simulink model "all_Challenges_all_controllers_slrd"  (R2024a)
settings: Solver=FixedStepAuto  StartTime=0.0  StopTime=inf  RelTol=1e-3  EnableMultiTasking=on
model workspace (MATLAB code in the model file):
  | num_pol_pairs = 7;
  | res_period = 5000;
  | res_pwm   = 2^8;
  | 
  | whl.rad = 0.045;
  | axle.length=0.18;
undefined symbols (not defined in the file): DiscIntNeverNeededParam
libraries: MecRoKa_SFunction_Library x20, slpidlib x5, simulink x4
(part 2 of 2)

== system all_Challenges_all_controllers_slrd/state control/do_BLDC_control.my_control_BLDC2/Task3/Subsystem ==
  Input : Inport
  Inport : Inport  Port=2
  Sum : Sum  Inputs=-+
  Output : Outport
  wires:
  Sum/1 -> Output/1
  Inport/1 -> Sum/1
  Input/1 -> Sum/2

== stateflow chart all_Challenges_all_controllers_slrd/state control ==
  state system_off
    en, du: phi_dot_left   = double(0.0);
    en, du: phi_dot_right = double(0.0);
    en, du: BLDC_on_flag = false;
  state do_BLDC_control
    en, du: BLDC_on_flag = true;
    en, du : [phi_dot_left, phi_dot_right,position_x,yaw_pos,Yaw_rate]=my_control_BLDC2(pitch_est, pitch_rate_est, vel_trgt, yaw_rate_trgt,position_trg,yaw_rate,control_switch,gain_switch);
    state [phi_dot_left1,phi_dot_right1,position_x,yaw_pos,Yaw_rate] = my_control_BLDC2(pitch_est1,pitch_rate_est_in1,vel_trgt_in1,yaw_rate_trgt_in,position_trg,yaw_rate,control_switch,gain_switch) [function]
  (default) -> system_off
  system_off -> do_BLDC_control : [op_mode ~= 0 ]
  do_BLDC_control -> system_off : [op_mode == 0 ]
  data: pitch_est1 function_input double size=1; pitch_rate_est_in1 function_input double size=1; vel_trgt_in1 function_input double size=1; yaw_rate_trgt_in function_input double size=1; phi_dot_left1 function_output double size=1; phi_dot_right1 function_output double size=1; position_trg function_input double size=1; position_x function_output; yaw_rate function_input double size=1; yaw_pos function_output; control_switch function_input double size=1; Yaw_rate function_output; gain_switch function_input double size=1; BLDC_on_flag output boolean; yaw_rate_trgt input double size=1; vel_trgt input double size=1; op_mode input uint8; pitch_est input double size=1; pitch_rate_est input double size=1; phi_dot_right output; phi_dot_left output; position_x output; position_trg input; yaw_rate input; yaw_pos output; control_switch input; Yaw_rate output; gain_switch input
  events: t_fc_state_ctrl input FUNCTION_CALL_EVENT

== stateflow chart all_Challenges_all_controllers_slrd/target mix logic ==
  state disarmed
    en, du: op_mode = uint8(0);
    en, du: vel_trgt = 0;
    en, du: yaw_rate_trgt  = 0;
  state armed
    en, du: op_mode = operation_mode;
    en, du: yaw_rate_trgt  = yaw_rate_trgt_auto;
    state autonomous
      en, du: vel_trgt   = vel_trgt_auto;
    (default) -> (junction 18)
    (junction 18) -> autonomous
  (default) -> (junction 15)
  (junction 15) -> armed [order 1] : [armed_flag == true]
  (junction 15) -> disarmed [order 2]
  disarmed -> armed : [armed_flag == true]
  armed -> disarmed : [armed_flag == false]
  data: yaw_rate_trgt output double size=1; vel_trgt output double size=1; armed_flag input boolean size=1; operation_mode input uint8 size=1; vel_trgt_auto input double size=1; yaw_rate_trgt_auto input double size=1; op_mode output uint8
  events: t_fc_trgt_mix_logic input FUNCTION_CALL_EVENT

== stateflow chart all_Challenges_all_controllers_slrd/attitude  estimation ==
  state do_state_estimation
    en: cut_off_freq = 1.;
    en: step_size = get_dt();
    en: [pitch_est, pitch_rate_est,yaw_rate] = estimate_angulars_script(double(acc_gyro_meas(2)), double(acc_gyro_meas(3)), double(acc_gyro_meas(4)),double(acc_gyro_meas(6)),cut_off_freq, step_size );
    state dt = get_dt [function]
    state [pit_est,pit_rate_est] = estimate_angulars_graph(acc_forward_neas,acc_verical_meas,pitch_rate_meas,fc,dt) [function]
  (default) -> do_state_estimation
  do_state_estimation -> do_state_estimation
  data: dt function_output; acc_forward_neas function_input double size=1; acc_verical_meas function_input double size=1; pit_est function_output double; pitch_rate_meas function_input double size=1; pit_rate_est function_output double; fc function_input double size=1; dt function_input double size=1; acc_forward_meas function_input; acc_vertical_meas function_input; pitch_rate_meas function_input; yaw_rate_raw function_input; pit_est function_output; pit_rate_est function_output; fc function_input; dt function_input; yaw_rate function_output; pitch_est output double size=1; pitch_rate_est output double size=1; acc_gyro_meas input int32 size=6; cut_off_freq local; step_size local double size=1; yaw_rate output
  events: t_fc_state_est input FUNCTION_CALL_EVENT
  function [pit_est, pit_rate_est,yaw_rate] = estimate_angulars_script(acc_forward_meas, acc_vertical_meas, pitch_rate_meas, yaw_rate_raw, fc, dt):
    | function [pit_est, pit_rate_est,yaw_rate] = estimate_angulars_script(acc_forward_meas, acc_vertical_meas, pitch_rate_meas, yaw_rate_raw, fc, dt)
    | % created by GBi 14.05.2020
    | % complementary filter combines high (HP) and low pass (LP) filter 
    | % signals with the same cutoff-frequency fc
    | %
    | % transfer function for LP: 1/(tau*s+1)
    | % transfer function for HP: tau*s/(tau*s+1)
    | % combining a HP with an integration (multiply with 1/s) yields: tau/(tau*s+1)
    | %
    | % first order approximation with time step size dt yields
    | % for LP:               new_value = C*old_value +(1-C)*actual_value
    | % for HP + integration: new_value = C*(old_value + delta_t*actual_value)
    | % with constant C = tau/(tau+dt)
    | %
    | % with cutoff angular frequency omega_c=1/tau and omega_c=2*pi*fc
    | % tau = 1./(2*pi*fc)
    | %
    | % complementry filter here combines LP filtered pitch estimation
    | % based on accelerometer data and integrated HP filtered pitch estimation
    | % based on gyro data
    | %
    | %----------------------------------------------------------------------------
    | persistent tau C pitch_from_acc_LP_filtered pitch_from_gyro_HP_filtered
    | if isempty(tau);
    |     tau = 1./ (2*pi*fc);
    |     C = tau/(tau+dt);
    |     pitch_from_acc_LP_filtered = 0.0;
    |     pitch_from_gyro_HP_filtered = 0.0;
    | end 
    | pitch_from_acc = atan2(acc_forward_meas, acc_vertical_meas);
    | pit_rate_est = pitch_rate_meas*pi/18000; %result in [rad/s]
    | pitch_from_acc_LP_filtered  = C*pitch_from_acc_LP_filtered +(1-C)*pitch_from_acc;
    | pitch_from_gyro_HP_filtered = C*(pitch_from_gyro_HP_filtered+pit_rate_est*dt);
    | pit_est = pitch_from_acc_LP_filtered + pitch_from_gyro_HP_filtered; %result in [rad]
    | yaw_rate = yaw_rate_raw*pi/18000;

== stateflow chart all_Challenges_all_controllers_slrd/mode set logic ==
  state set_actual_mode
    state set_autonomous_targets
      en: armed_flag = true;
      en: operation_mode = uint8(Dip_switch);
      state op_mode =Dip_switch [function]
    state swich_off_if_high_pitch
      en: operation_mode = uint8(0);
    (default) -> (junction 22)
    (junction 22) -> swich_off_if_high_pitch [order 1] : [abs(pitch_actual)>50*2*pi/360]
    (junction 22) -> set_autonomous_targets [order 2]
    swich_off_if_high_pitch -> set_actual_mode
    set_autonomous_targets -> set_actual_mode
  (default) -> set_actual_mode
  data: op_mode function_output; armed_flag output boolean size=1; operation_mode output uint8 size=1; pitch_actual input double size=1
  events: t_fc_mode_set_logic input FUNCTION_CALL_EVENT

== matlab function all_Challenges_all_controllers_slrd/mode set logic/set_actual_mode.set_autonomous_targets.Dip_switch/Truth Table ==
  data: A1 input; y output; A3 input; A2 input; A4 input
function y = fcn(A1, A3, A2, A4)

aVarTruthTableCondition_1 = false;
aVarTruthTableCondition_2 = false;
aVarTruthTableCondition_3 = false;
aVarTruthTableCondition_4 = false;


% Dip_Switch_1

aVarTruthTableCondition_1 = logical(A1>=4.9);

% Dip_Switch_2

aVarTruthTableCondition_2 = logical(A2>=4.9);

% Dip_Switch_3

aVarTruthTableCondition_3 = logical(A3>=4.9);

% Dip_Switch_4

aVarTruthTableCondition_4 = logical(A4>= 4.9);

if (aVarTruthTableCondition_1 && ~aVarTruthTableCondition_2 && ~aVarTruthTableCondition_3 && ~aVarTruthTableCondition_4)
    aFcnTruthTableAction_1();
elseif (~aVarTruthTableCondition_1 && aVarTruthTableCondition_2 && ~aVarTruthTableCondition_3 && ~aVarTruthTableCondition_4)
    aFcnTruthTableAction_2();
elseif (~aVarTruthTableCondition_1 && ~aVarTruthTableCondition_2 && aVarTruthTableCondition_3 && ~aVarTruthTableCondition_4)
    aFcnTruthTableAction_3();
elseif (~aVarTruthTableCondition_1 && ~aVarTruthTableCondition_2 && ~aVarTruthTableCondition_3 && aVarTruthTableCondition_4)
    aFcnTruthTableAction_4();
else % Default
    aFcnTruthTableAction_5();
end

function aFcnTruthTableAction_1()

% Challenge_1

y = 2;

function aFcnTruthTableAction_2()

% Challenge_2

y=3

function aFcnTruthTableAction_3()

% Challenge_3

y=4

function aFcnTruthTableAction_4()

% Challenge_4

y = 5;

function aFcnTruthTableAction_5()

% default

y=1

== stateflow chart all_Challenges_all_controllers_slrd/autonomous targets ==
  state set_autonomous_targets
    state Op_mode_steady_balancing_1
      en, du: vel_trgt_auto   = 0.00;
      en, du: yaw_rate_trgt_auto  = 0.0;
    state Challenge_1_drive_fast
      en, du: gain_sw  = 2;
      state stop1
        en, du: vel_trgt_auto   = 0.00;
        en, du: yaw_rate_trgt_auto  = 0.0;
        en, du: position_trg = 0;
        en, du: Ctrl_SW  = 1;
      state Initial_acc
        en, du: vel_trgt_auto   = 1;
        en, du: yaw_rate_trgt_auto  = 0;
        en, du: position_trg = 2.8;
        en, du: Ctrl_SW  = 1;
      state Constant_speed
        en, du: vel_trgt_auto   = 1.5;
        en, du: yaw_rate_trgt_auto  = 0.0;
        en, du: position_trg = 0;
        en, du: Ctrl_SW  = 1;
      state stop
        en, du: vel_trgt_auto   = 0.0;
        en, du: yaw_rate_trgt_auto  = 0.0;
        en, du: position_trg = 0;
        en, du: Ctrl_SW  = 4;
      (default) -> set_autonomous_targets.Challenge_1_drive_fast.stop1
      set_autonomous_targets.Challenge_1_drive_fast.stop1 -> Initial_acc : after(3,sec)
      Initial_acc -> Constant_speed : after(1.8,sec)
      Constant_speed -> stop : after(9,sec)
      stop -> Challenge_1_drive_fast : after(2.5,sec)
    state Challenge_2
      en, du: gain_sw  = 1;
      state Turn1
        en, du: vel_trgt_auto   = 0.0;
        en, du: yaw_rate_trgt_auto  = pi;
        en, du: Ctrl_SW  = 1;
        en, du: gain_sw  = 1;
      state turn2
        en, du: vel_trgt_auto   = 0.0;
        en, du: yaw_rate_trgt_auto  = pi;
        en, du: Ctrl_SW  = 1;
        en, du: gain_sw  = 1;
      state stop1
        en, du: vel_trgt_auto   = 0.00;
        en, du: yaw_rate_trgt_auto  = 0.0;
        en, du: position_trg = 0;
        en, du: Ctrl_SW  = 2;
        en, du: gain_sw  = 1;
      state Go_forward1
        en, du: vel_trgt_auto   = 0.00;
        en, du: yaw_rate_trgt_auto  = 0.0;
        en, du: position_trg = 1;
        en, du: Ctrl_SW  = 2;
      state go_forward3
        en, du: vel_trgt_auto   = 0.0;
        en, du: yaw_rate_trgt_auto  = 0.0;
        en, du: position_trg = 3;
        en, du: Ctrl_SW  = 2;
        en, du: gain_sw  = 1;
      state stop4
        en, du: vel_trgt_auto   = 0.00;
        en, du: yaw_rate_trgt_auto  = 0.0;
        en, du: position_trg = 2;
        en, du: Ctrl_SW  = 2;
        en, du: gain_sw  = 1;
      state turn3
        en, du: vel_trgt_auto   = 0.0;
        en, du: yaw_rate_trgt_auto  = pi;
        en, du: Ctrl_SW  = 1;
        en, du: gain_sw  = 1;
      state turn4
        en, du: vel_trgt_auto   = 0.0;
        en, du: yaw_rate_trgt_auto  = pi;
        en, du: Ctrl_SW  = 1;
        en, du: gain_sw  = 1;
      turn2 -> stop4 : [yaw_pos>2*pi-0.25]
      Go_forward1 -> Turn1 : [position_x>=1&&after(2.5,sec)]
      (default) -> set_autonomous_targets.Challenge_2.stop1
      Turn1 -> turn2 : [yaw_pos>pi-0.25]
      set_autonomous_targets.Challenge_2.stop1 -> Go_forward1 : after(3,sec)
      turn4 -> go_forward3 : [yaw_pos>4*pi-0.25]
      turn3 -> turn4 : [yaw_pos>3*pi-0.25]
      stop4 -> turn3 : [position_x>=1.9&&after(2.5,sec)]
    state Op_mode_fast_mode
      en, du: Ctrl_SW  = 5;
      en, du: gain_sw  = 3;
      state stop1
        en, du: vel_trgt_auto   = 0.00;
        en, du: yaw_rate_trgt_auto  = 0.0;
        en, du: position_trg= 0.0;
      state Go
        en, du: vel_trgt_auto  = 00;
        en, du: yaw_rate_trgt_auto  = 0.0;
        en, du: position_trg= 0;
      state stop2
        en, du: vel_trgt_auto   = 0.0;
        en, du: yaw_rate_trgt_auto  = 0.0;
        en, du: position_trg= 0;
      (default) -> set_autonomous_targets.Op_mode_fast_mode.stop1
      set_autonomous_targets.Op_mode_fast_mode.stop1 -> Go : [after(5,sec)]
      Go -> stop2 : [after(60,sec)]
    state Challenge_4_Figure_8
      en, du: Ctrl_SW  = 3;
      en, du: gain_sw  = 4;
      state cal
        en, du: vel_trgt_auto   = 0.00;
        en, du: yaw_rate_trgt_auto  = 0.0;
        en, du: position_trg = 0;
      state forward1m
        en, du: vel_trgt_auto   = 0.5;
        en, du: yaw_rate_trgt_auto  = yaw_rate;
        en, du: position_trg = 1.9;
      state forward1m3
        en, du: vel_trgt_auto   = 0.5;
        en, du: yaw_rate_trgt_auto  =yaw_rate;
        en, du: position_trg = 3.4;
      state forward1m7
        en, du: vel_trgt_auto   = 0.6;
        en, du: yaw_rate_trgt_auto  =-yaw_rate;
        en, du: position_trg = 1.57/2+3.14+0.3;
      state forward1m6
        en, du: vel_trgt_auto   = 0.5;
        en, du: yaw_rate_trgt_auto  =-yaw_rate;
        en, du: position_trg = 5;
      state forward1m5
        en, du: vel_trgt_auto   = 0.7;
        en, du: yaw_rate_trgt_auto  =-yaw_rate;
        en, du: position_trg = 6.5;
      state forward1m8
        en, du: vel_trgt_auto   = 0.5;
        en, du: yaw_rate_trgt_auto  =0;
        en, du: position_trg = 6.6;
      (default) -> cal
      cal -> forward1m : [after(2,sec)]
      forward1m -> forward1m3 : [position_x>=1.57]
      forward1m3 -> forward1m7 : [position_x>=3.21]
      forward1m7 -> forward1m6 : [position_x>=1.57/2+3.14]
      forward1m6 -> forward1m5 : [position_x>=4.71]
      forward1m5 -> forward1m8 : [position_x>=6.35]
    state OP_mode_off_0
      en, du: vel_trgt_auto   = 0.00;
      en, du: yaw_rate_trgt_auto  = 0.0;
    (default) -> (junction 57)
    (junction 57) -> Op_mode_steady_balancing_1 [order 1] : [op_mode == 1 ]
    (junction 57) -> (junction 59) [order 2]
    (junction 59) -> (junction 58)
    (junction 58) -> (junction 61)
    (junction 61) -> Challenge_1_drive_fast [order 1] : [op_mode == 2]
    (junction 61) -> (junction 90) [order 2]
    (junction 90) -> Challenge_2 [order 1] : [op_mode == 3]
    (junction 90) -> (junction 102) [order 2]
    (junction 102) -> Op_mode_fast_mode [order 1] : [op_mode == 4]
    (junction 102) -> (junction 118) [order 2]
    (junction 118) -> Challenge_4_Figure_8 [order 1] : [op_mode == 5]
    (junction 118) -> (junction 62) [order 2]
    (junction 62) -> OP_mode_off_0
  (default) -> set_autonomous_targets
  data: op_mode input uint8 size=1; vel_trgt_auto output double size=1; yaw_rate_trgt_auto output double size=1; actphileft input; actphiright input; position_x input; position_trg output; yaw_pos input; Ctrl_SW output; yaw_rate input size=1; gain_sw output
  events: t_fc_auto_trgts input FUNCTION_CALL_EVENT
